simulink model "sl_quadrotor_guidance"  (R2022a)
settings: Solver=VariableStepAuto  StartTime=0.0  StopTime=10  MaxStep=0.1  RelTol=1e-3  EnableMultiTasking=on
PreLoadFcn:
  | % load parameters of the default quadrotor
  | disp('Quadrotor parameters loaded by PreLoadFcn')
  | mdl_quadrotor
StartFcn:
  | f = findall(groot,'Name','UAV Animation');
  | if (length(f) > 1)
  |    f = f(1);
  | end
  | 
  | % Fix plot axes limits
  | ax = f.findobj("Type", "Axes");
  | ax.ZLim = [0 6];
  | ax.XLim = [-5 5];
  | ax.YLim = [-5 5];
  | ax.XLabel.String = 'x';
  | ax.YLabel.String = 'y';
  | ax.ZLabel.String = 'z (height above ground)';
undefined symbols (not defined in the file or in its folder): rotm2d
libraries: robotcorelib x1, uavalgslib x1, uavutilslib x1, simulink x1
Description:
  | Closed-loop simulation of a quadrotor aerial robot.
  | Replaces the attitude controllers, control mixer, and dynamics simulation with a single
  | Guidance Model block.
  | 
  | Robotics, Vision and Control - 3rd Edition; Section 4.2
settings Model: Creator=corkep  LastModifiedBy=rpill
settings SolverCC: AlgebraicLoopSolver=TrustRegion  MaxZcPerStep=1
settings DataIOCC: LimitDataPoints=on  TimeSaveName=t  OutputSaveName=y
settings OptimizationCC: ExpressionDepthLimit=2147483647  LifeSpan=inf
settings DebuggingCC: UnderspecifiedInitializationDetection=Classic  MergeDetectMultiDrivingBlocksExec=none  SolverPrmCheckMsg=warning  UnconnectedInputMsg=warning  UnconnectedOutputMsg=warning  UnconnectedLineMsg=warning  AllowSymbolicDim=off  StateNameClashWarn=warning  SFUnexpectedBacktrackingDiag=warning  SFNoUnconditionalDefaultTransitionDiag=warning  SFExecutionAtInitializationDiag=none  SFMachineParentedDataDiag=warning  ArithmeticOperatorsInVariantConditions=warning
settings HardwareCC: ProdBitPerPointer=32  ProdBitPerSizeT=32  ProdBitPerPtrDiffT=32  ProdLargestAtomicFloat=None  ProdIntDivRoundTo=Undefined  ProdEndianess=Unspecified  ProdWordSize=32  ProdHWDeviceType=32-bit Generic
settings ModelReferenceCC: PropagateSignalLabelsOutOfModel=off
settings SFSimCC: SimUseLocalCustomCode=off  CustomCodeUndefinedFunction=UseInterfaceOnly
settings RTWCC: RTWUseLocalCustomCode=off  DLArmComputeVersion=19.05
settings CodeAppCC: StateflowObjectComments=on
settings GRTTargetCC: TargetLangStandard=C89/C90 (ANSI)  CombineOutputUpdateFcns=off  GRTInterface=on
settings ConfigComp: CovMetricSettings=dw  CovSaveCumulativeToWorkspaceVar=on  CovSaveSingleToWorkspaceVar=on  CovExternalEMLEnable=off  CovSFcnEnable=off

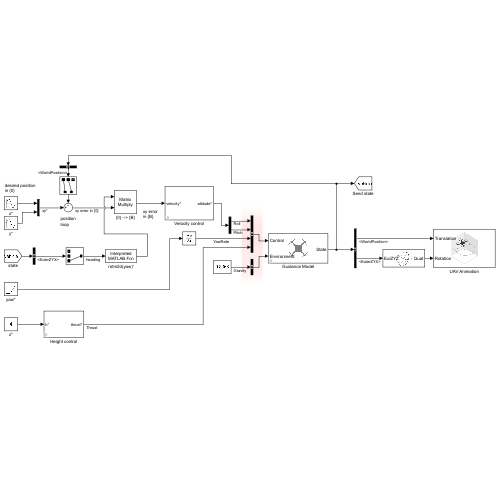
[thumbnail: Simulink's stored preview of the top-level diagram]
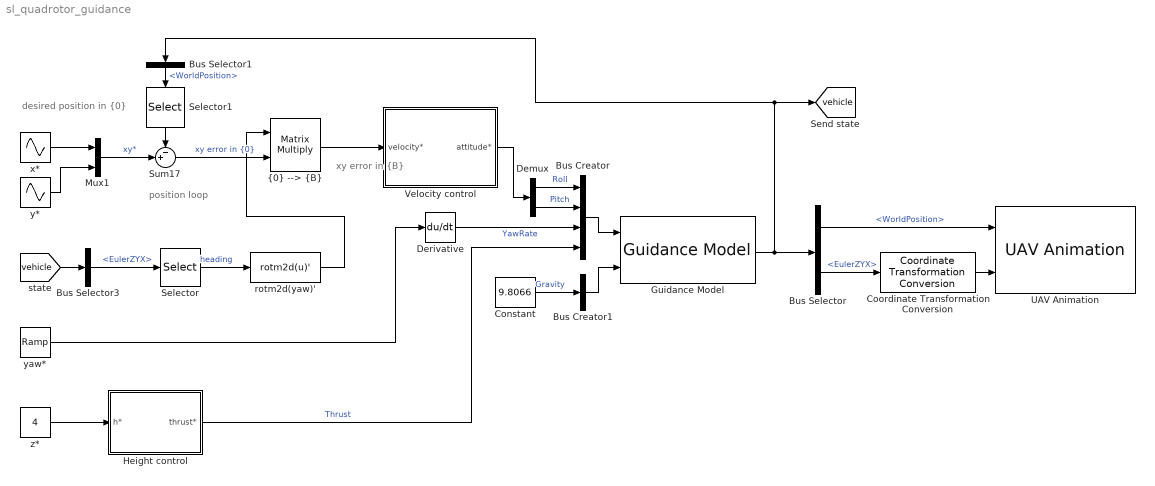
== system sl_quadrotor_guidance ==
  note: xy error
      | in {B}
  note: desired position
      | in {0}
  note: position
      | loop
  Bus Creator : BusCreator  Inputs=4  OutDataTypeStr=Bus: MultirotorGuidanceControlBus  NonVirtualBus=on
  Bus Creator1 : BusCreator  Inputs=1  OutDataTypeStr=Bus: MultirotorGuidanceEnvironmentBus  NonVirtualBus=on
  Bus Selector : BusSelector  OutputSignals=WorldPosition,EulerZYX
  Bus Selector1 : BusSelector  OutputSignals=WorldPosition
  Bus Selector3 : BusSelector  OutputSignals=EulerZYX
  Constant : Constant  Value=9.8066
  Coordinate Transformation Conversion : robotcorelib/Coordinate Transformation Conversion  InputRepresentation=Euler Angles  InputEulerSequence=ZYZ  ShowTrVecInputPort=on  OutputRepresentation=Quaternion  OutputEulerSequence=ZYX  ShowTrVecOutputPort=on  SimulateUsing=Interpreted execution
      settings: SourceProductBaseCode=RO,NV,RR,UV
  Demux : Demux  Outputs=2
  Derivative : Derivative
  Guidance Model : uavalgslib/Guidance Model  ModelType=MultirotorGuidance  SpecifiedDataType=double  SimulateUsing=Code generation  InitialWorldPositionMultirotor=[0; 0; 0]  InitialWorldVelocityMultirotor=[0; 0; 0]  InitialEulerZYXMultirotor=[0; 0; 0]  InitialBodyAngularRateRPYMultirotor=[0; 0; 0]  InitialThrustMultirotor=0  InitialNorthFixedWing=0  InitialEastFixedWing=0  InitialHeightFixedWing=0  InitialAirSpeedFixedWing=0  InitialHeadingAngleFixedWing=0  InitialFlightPathAngleFixedWing=0  InitialRollAngleFixedWing=0  InitialRollAngleRateFixedWing=0  PDRollMultirotor=[3402.97,116.67]  PDPitchMultirotor=[3402.97, 116.67]  PYawRateMultirotor=1950  PThrustMultirotor=3900  MassMultirotor=0.1  PHeightFixedWing=3.9  PHeadingAngleFixedWing=3.9  PFlightPathAngleFixedWing=39  PDRollFixedWing=[3402.97, 116.67]  PAirSpeedFixedWing=1  FlightPathAngleLimitsFixedWing=[-pi/2, pi/2]  StateBusName='MultirotorGuidanceStateBus'  ControlBusName='MultirotorGuidanceControlBus'  EnvironmentBusName='MultirotorGuidanceEnvironmentBus'  DataType=double
      settings: SourceProductBaseCode=UV
  Height control : Subsystem  mask{P=4, D=1, T0=40}
      mask prompts: P "Proportional gain"; D "Derivative gain"; T0 "Thrust feedforward"
  Mux1 : Mux  Inputs=2
  Selector : Selector  InputPortWidth=3  IndexOptions=Index vector (dialog)  Indices=[3]  OutputSizes=1
  Selector1 : Selector  InputPortWidth=3  IndexOptions=Index vector (dialog)  Indices=[1 2]  OutputSizes=1
  Sum17 : Sum  Inputs=-+|  OutDataTypeStr=Inherit: Inherit via back propagation
  UAV Animation : uavutilslib/UAV Animation  UAVType=Multirotor  UAVSize=2  InertialZDirection=Down  SampleTime=0.1
      settings: SourceProductBaseCode=UV
  Velocity control : Subsystem  mask{P=0.1, D=2}
      mask prompts: P "Proportional gain"; D "Derivative gain"
  rotm2d(yaw)' : MATLABFcn  MATLABFcn=rotm2d(u)'  OutputDimensions=[2 2]  Output1D=off
  x* : Sin  Amplitude=3  Frequency=2*pi*.125  Phase=-pi/2  SampleTime=0
  y* : Sin  Amplitude=3  Frequency=2*pi*.125  SampleTime=0
  yaw* : simulink/Sources/Ramp  slope=0.2  start=2  InitialOutput=0
  z* : Constant  Value=4  SampleTime=0
  "{0} --> {B}" : Product  Multiplication=Matrix(*)  RndMeth=Zero
  tag scope: vehicle=global
  wires:
  x*/1 -> Mux1/1
  y*/1 -> Mux1/2
  Sum17/1 -> "{0} --> {B}"/2  "xy error in {0}"
  "{0} --> {B}"/1 -> Velocity control/1(velocity*)
  Velocity control/1(attitude*) -> Demux/1
  z*/1 -> Height control/1(h*)
  Mux1/1 -> Sum17/2  "xy*"
  rotm2d(yaw)'/1 -> "{0} --> {B}"/1
  Height control/1(thrust*) -> Bus Creator/4  "Thrust"
  Coordinate Transformation Conversion/1 -> UAV Animation/2
  Demux/1 -> Bus Creator/1  "Roll"
  Demux/2 -> Bus Creator/2  "Pitch"
  Derivative/1 -> Bus Creator/3  "YawRate"
  Bus Creator/1 -> Guidance Model/1
  Guidance Model/1 -> Bus Selector/1, [vehicle], Bus Selector1/1
  yaw*/1 -> Derivative/1
  [vehicle] -> Bus Selector3/1
  Bus Selector/1 -> UAV Animation/1  "<WorldPosition>"
  Bus Selector/2 -> Coordinate Transformation Conversion/1  "<EulerZYX>"
  Bus Selector3/1 -> Selector/1  "<EulerZYX>"
  Selector/1 -> rotm2d(yaw)'/1  "heading"
  Bus Selector1/1 -> Selector1/1  "<WorldPosition>"
  Selector1/1 -> Sum17/1
  Constant/1 -> Bus Creator1/1  "Gravity"
  Bus Creator1/1 -> Guidance Model/2

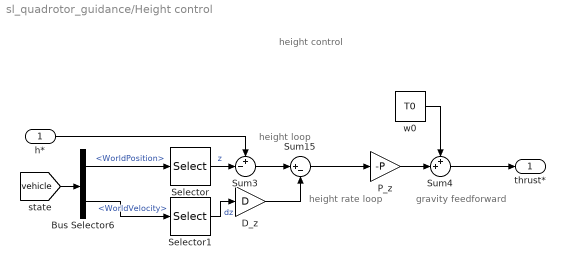
== system sl_quadrotor_guidance/Height control ==
  note: height control
  note: gravity feedforward
  note: height rate
      | loop
  note: height
      | loop
  h* : Inport
  Bus Selector6 : BusSelector  OutputSignals=WorldPosition,WorldVelocity
  D_z : Gain  Gain=D
  P_z : Gain  Gain=-P
  Selector : Selector  InputPortWidth=3  IndexOptions=Index vector (dialog)  Indices=[3]  OutputSizes=1
  Selector1 : Selector  InputPortWidth=3  IndexOptions=Index vector (dialog)  Indices=[3]  OutputSizes=1
  Sum15 : Sum  Inputs=|+-
  Sum3 : Sum  Inputs=+-|
  Sum4 : Sum  Inputs=++|
  w0 : Constant  Value=T0  SampleTime=0
  thrust* : Outport
  wires:
  w0/1 -> Sum4/1
  Sum15/1 -> P_z/1
  P_z/1 -> Sum4/2
  h*/1 -> Sum3/1
  Sum3/1 -> Sum15/1
  D_z/1 -> Sum15/2
  Sum4/1 -> thrust*/1
  [vehicle] -> Bus Selector6/1
  Bus Selector6/1 -> Selector/1  "<WorldPosition>"
  Selector/1 -> Sum3/2  "z"
  Bus Selector6/2 -> Selector1/1  "<WorldVelocity>"
  Selector1/1 -> D_z/1  "dz"

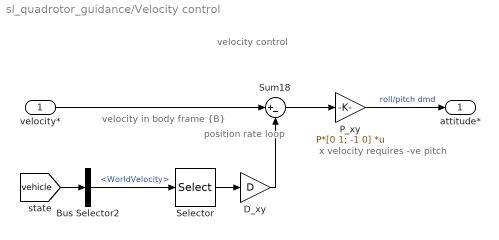
== system sl_quadrotor_guidance/Velocity control ==
  note: x velocity requires -ve pitch
  note: velocity in body frame {B}
  note: velocity control
  note: position rate
      | loop
  velocity* : Inport
  Bus Selector2 : BusSelector  OutputSignals=WorldVelocity
  D_xy : Gain  Gain=D
  P_xy : Gain  Gain=P*[0 1; -1 0]  Multiplication=Matrix(K*u)
  Selector : Selector  InputPortWidth=3  IndexOptions=Index vector (dialog)  Indices=[1 2]  OutputSizes=1
  Sum18 : Sum  Inputs=|+-
  attitude* : Outport
  wires:
  D_xy/1 -> Sum18/2
  Sum18/1 -> P_xy/1
  velocity*/1 -> Sum18/1
  [vehicle] -> Bus Selector2/1
  P_xy/1 -> attitude*/1  "roll/pitch dmd"
  Bus Selector2/1 -> Selector/1  "<WorldVelocity>"
  Selector/1 -> D_xy/1
